simulink subsystem "rocket_plant_combined"  (R2024b)
settings: Solver=VariableStepAuto  StartTime=0.0  StopTime=10.0  RelTol=1e-3
settings Model: Creator=joedo  LastModifiedBy=finnb

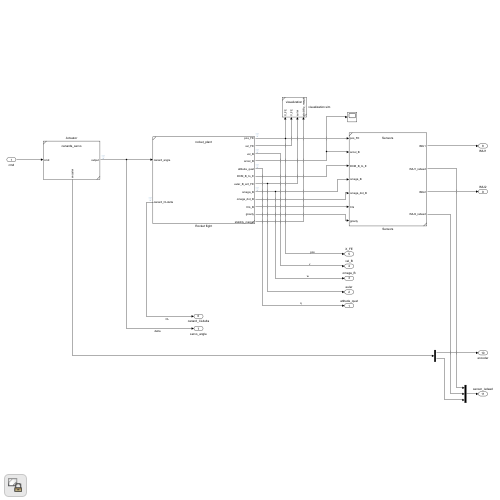
[thumbnail: Simulink's stored preview of the top-level diagram]
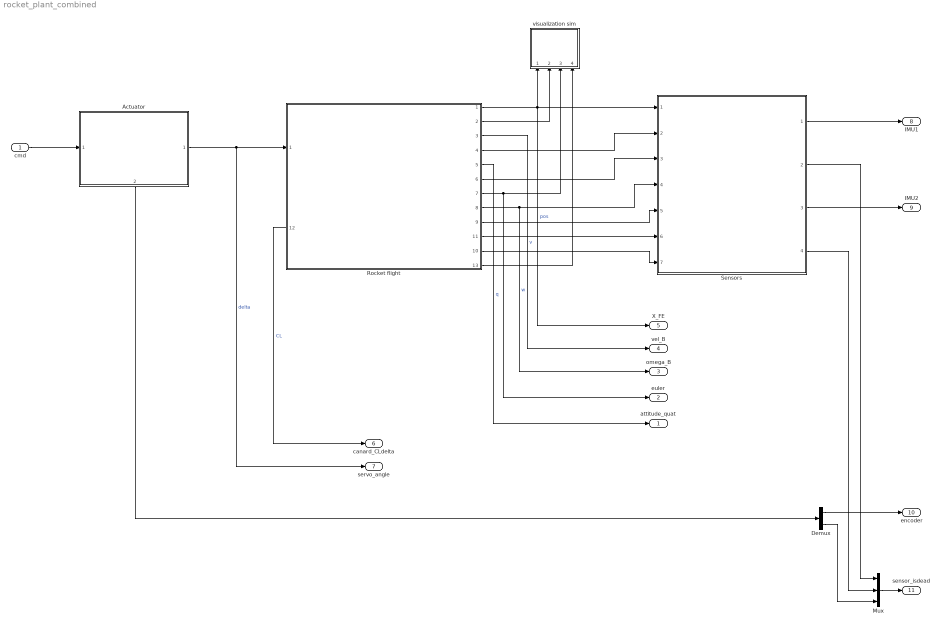
== system rocket_plant_combined ==
  cmd : Inport
  Actuator : Subsystem  ReferencedSubsystem=canards_servo
      settings: PortSchema="{\"entries\":[{\"content\":{\"sides\":[{\"content\":{\"connectorIds\":[\"In1\"]},\"type\":\"ConnectorPlacement.EquallySpacedRectSide\",\"uuid\":\"f1fe2692-4f3a-49f6-a037-219451f9c8a9\"},{\"content\":{\"connectorIds\":[\"Out1\"],\"side\":\"RIGHT\"},\"type\":\"ConnectorPlacement.EquallySpacedRectSide\",\"uuid\":\"c09abda5-ce02-4dc4-8bf7-df22ff98c510\"},{\"content\":{\"side\":\"TOP\"},\"type\":\"ConnectorPlacement.EquallySpacedRectSide\",\"uuid\":\"d89775cf-018a-424b-8fdc-70f841ad885b\"},{\"content\":{\"connectorIds\":[\"Out2\"],\"side\":\"BOTTOM\"},\"type\":\"ConnectorPlacement.EquallySpacedRectSide\",\"uuid\":\"dc16bf3c-a1ac-4f88-a587-41692023e4d4\"}]},\"type\":\"ConnectorPlacement.EquallySpacedConnector\",\"uuid\":\"f43e876a-9b83-427e-9fa5-752c9eee6ca7\"}],\"packageUris\":[\"http://schema.mathworks.com/mf0/Connector/R2020b\"],\"version\":\"1.0\"}"
  Demux : Demux  Outputs=[1 1]
  Mux : Mux  Inputs=3
  Rocket flight : Subsystem  ReferencedSubsystem=rocket_flight
      settings: PortSchema="{\"entries\":[{\"content\":{\"sides\":[{\"content\":{\"connectorIds\":[\"In1\",\"Out12\"]},\"type\":\"ConnectorPlacement.EquallySpacedRectSide\",\"uuid\":\"9f79cae0-15ae-41cc-86ca-52b2ba536b20\"},{\"content\":{\"connectorIds\":[\"Out1\",\"Out2\",\"Out3\",\"Out4\",\"Out5\",\"Out6\",\"Out7\",\"Out8\",\"Out9\",\"Out11\",\"Out10\",\"Out13\"],\"side\":\"RIGHT\"},\"type\":\"ConnectorPlacement.EquallySpacedRectSide\",\"uuid\":\"ebcb1700-a632-4dda-8ea5-5b87e6fa3b6a\"},{\"content\":{\"side\":\"TOP\"},\"type\":\"ConnectorPlacement.EquallySpacedRectSide\",\"uuid\":\"efdf61b2-36e8-47a1-89a6-5eee4bf93d92\"}]},\"type\":\"ConnectorPlacement.EquallySpacedConnector\",\"uuid\":\"49b511cd-3c57-4668-a103-5fb675f3d38c\"}],\"packageUris\":[\"http://schema.mathworks.com/mf0/Connector/R2020b\"],\"version\":\"1.0\"}"
  Sensors : Subsystem  ReferencedSubsystem=Sensors
  visualization sim : Subsystem  ReferencedSubsystem=visualization
  attitude_quat : Outport
  euler : Outport  Port=2
  omega_B : Outport  Port=3
  vel_B : Outport  Port=4
  X_FE : Outport  Port=5
  canard_CLdelta : Outport  Port=6
  servo_angle : Outport  Port=7
  IMU1 : Outport  Port=8
  IMU2 : Outport  Port=9
  encoder : Outport  Port=10
  sensor_isdead : Outport  Port=11
  wires:
  Rocket flight/11 -> Sensors/6
  Rocket flight/7 -> euler/1, visualization sim/3
  Rocket flight/1 -> visualization sim/1, Sensors/1, X_FE/1  "pos"
  Actuator/1 -> servo_angle/1, Rocket flight/1  "delta"
  Rocket flight/5 -> attitude_quat/1  "q"
  Rocket flight/9 -> Sensors/5
  Rocket flight/8 -> omega_B/1, Sensors/4  "w"
  Rocket flight/4 -> Sensors/2
  Rocket flight/6 -> Sensors/3
  Rocket flight/10 -> Sensors/7
  Rocket flight/3 -> vel_B/1  "v"
  Rocket flight/2 -> visualization sim/2
  Sensors/1 -> IMU1/1
  Sensors/3 -> IMU2/1
  cmd/1 -> Actuator/1
  Actuator/2 -> Demux/1
  Rocket flight/12 -> canard_CLdelta/1  "CL"
  Rocket flight/13 -> visualization sim/4
  Mux/1 -> sensor_isdead/1
  Sensors/2 -> Mux/1
  Sensors/4 -> Mux/2
  Demux/1 -> encoder/1
  Demux/2 -> Mux/3
